simulink model "lag3options"  (R2018b)
settings: Solver=VariableStepAuto  StartTime=0.0  StopTime=10.0  RelTol=1e-3
settings Model: Creator=art58  LastModifiedBy=art58

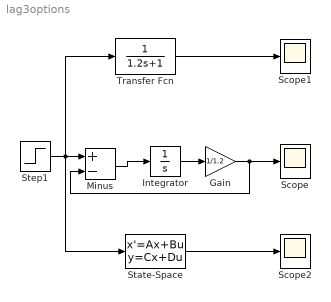
== system lag3options ==
  Gain : Gain  Gain=1/1.2
  Integrator : Integrator
  Minus : Sum  Inputs=+-
  Scope : Scope
  Scope1 : Scope
  Scope2 : Scope
  State-Space : StateSpace  A=-1/1.2  B=1/1.2  D=0  InitialCondition=0
  Step1 : Step  After=1.0  SampleTime=0
  Transfer Fcn : TransferFcn  Denominator=[1.2 1]
  wires:
  Step1/1 -> State-Space/1, Transfer Fcn/1, Minus/1
  Minus/1 -> Integrator/1
  Integrator/1 -> Gain/1
  Transfer Fcn/1 -> Scope1/1
  State-Space/1 -> Scope2/1
  Gain/1 -> Scope/1, Minus/2
